simulink model "Multibody_Street_Drone"  (R2019b)
settings: Solver=FixedStepAuto  StartTime=0.0  StopTime=20  FixedStep=0.0075  MaxStep=1e-1  MinStep=1e-7  RelTol=1e-3  AbsTol=1e-6
values from neighbouring files (symbols this model uses):
  Rear_brake = [0 1.82218650851 3.8277518469 5.98774429698 7.94202318038 9.84492098434 11.9533431061 13.8561462856 16.0160441112 18.021704074 19.9760775819 21.9303564653 ... (72 elements, 36x2)]    [Rear_brake.mat]
  TPS_0 = [469.425704648 608.284708657 814.443475346 1022.3060335 1213.13067704 1420.75786613 1608.14616582 1820.50021131 2024.31741075 2213.1951296 2423.41496358 2611.22557668 ... (88 elements, 44x2)]    [TPS_0.mat]
undefined symbols (not defined in the file or in its folder): Front_brake, sigbuilder_block, X, Y, Z
libraries: sm_lib x290, nesl_utility x136, simulink x2
(part 1 of 12)
settings Model: Creator=prave  LastModifiedBy=prave
settings SolverCC: AutoScaleAbsTol=off  MaxConsecutiveMinStep=2  ZeroCrossAlgorithm=Adaptive  AlgebraicLoopSolver=LineSearch
settings DataIOCC: ReturnWorkspaceOutputs=off
settings DebuggingCC: IgnoredZcDiagnostic=none

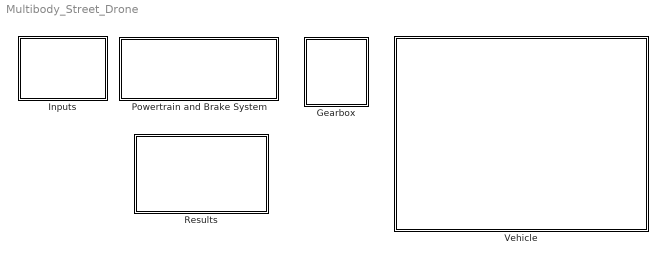
== system Multibody_Street_Drone ==
  Gearbox : Subsystem
  Inputs : Subsystem
  Powertrain and Brake System : Subsystem
  Results : Subsystem
  Vehicle : Subsystem

== system Multibody_Street_Drone/Gearbox ==
  For_reverse : Gain  Gain=-1
  Manual Switch1 : ManualSwitch  CurrentSetting=0
  Manual Switch2 : ManualSwitch
  Neutral : Constant  Value=0
  tag scope: tau=global
  wires:
  Manual Switch1/1 -> [tau]
  Neutral/1 -> Manual Switch1/1
  [final_tau] -> For_reverse/1, Manual Switch2/1
  Manual Switch2/1 -> Manual Switch1/2
  For_reverse/1 -> Manual Switch2/2

== system Multibody_Street_Drone/Inputs ==
  Delta : Subsystem
  Velocity : Subsystem

== system Multibody_Street_Drone/Powertrain and Brake System ==
  Abs : Abs
  Brake_system : Subsystem
  Divide : Product  Inputs=/*
  Driveline_viscous_losses : Subsystem
  Driver : simulink/Continuous/PID Controller  Controller=PID  Form=Parallel  TimeDomain=Continuous-time  SampleTime=-1  IntegratorMethod=Forward Euler  FilterMethod=Forward Euler  ControllerParametersSource=internal  P=150  I=1  D=0  UseFilter=on  N=100  TunerSelectOption=Transfer Function Based (PID Tuner App)  InitialConditionSource=internal  InitialConditionForIntegrator=0  InitialConditionForFilter=0  DifferentiatorICPrevScaledInput=0  ExternalReset=none  TrackingMode=off  Kt=1  LimitOutput=off  UpperSaturationLimit=inf  LowerSaturationLimit=-inf  LinearizeAsGain=on  AntiWindupMode=none  Kb=1  POutMin=[]  POutMax=[]  IOutMin=[]  IOutMax=[]  DOutMin=[]  DOutMax=[]  NOutMin=[]  NOutMax=[]  SumOutMin=[]  SumOutMax=[]  SaturationOutMin=[]  SaturationOutMax=[]  PParamMin=[]  PParamMax=[]  IParamMin=[]  IParamMax=[]  DParamMin=[]  DParamMax=[]  NParamMin=[]  NParamMax=[]  KbParamMin=[]  KbParamMax=[]  KtParamMin=[]  KtParamMax=[]  KbOutMin=[]  KbOutMax=[]  KtOutMin=[]  KtOutMax=[]  IntegratorOutMin=[]  IntegratorOutMax=[]  FilterOutMin=[]  FilterOutMax=[]  SumI1OutMin=[]  SumI1OutMax=[]  SumI2OutMin=[]  SumI2OutMax=[]  SumI3OutMin=[]  SumI3OutMax=[]  SumI4OutMin=[]  SumI4OutMax=[]  SumDOutMin=[]  SumDOutMax=[]  DifferentiatorOutMin=[]  DifferentiatorOutMax=[]  FilterDiffOutCoefMin=[]  FilterDiffOutCoefMax=[]  ReciprocalOutMin=[]  ReciprocalOutMax=[]  SumDenOutMin=[]  SumDenOutMax=[]  SumNumOutMin=[]  SumNumOutMax=[]  DivideOutMin=[]  DivideOutMax=[]  IntegratorContinuousStateAttributes=''  IntegratorStateMustResolveToSignalObject=off  IntegratorRTWStateStorageClass=Auto  FilterContinuousStateAttributes=''  FilterStateMustResolveToSignalObject=off  FilterRTWStateStorageClass=Auto  ParallelPVariant=InternalParameters  IdealPVariant=Disabled  IVariant=InternalParameters  DVariant=InternalParameters  IntegratorVariant=Continuous  SatVariant=Disabled  AWVariant=Passthrough  PCopyVariant=Disabled  TRVariant=Disabled  FdbkBlocksVariant=Forward  IdealPFdbkVariant=Disabled  SatFdbkVariant=Disabled  DerivativeFilterVariant=ContFilter  NVariant=InternalParameters  NCopyVariant=Disabled  FilterICVariant=InternalICsFilter  IntegratorICVariant=InternalICs  ExternalResetVariant=Disabled  TRSumVariant=Passthrough  SumFdbkVariant=Disabled  SumVariant=Sum_PID
  Gain1 : Gain  Gain=0.5
  Gear_ratio : Gain  Gain=9.23
  Motor : Subsystem
  Rate Limiter6 : RateLimiter  RisingSlewLimit=600  FallingSlewLimit=-1000  SampleTimeMode=inherited
  Scaling : Subsystem
  Scope : Scope
  Scope18 : Scope  NumInputPorts=2
  Subtract : Sum  Inputs=+-
  Subtract2 : Sum  Inputs=+-
  To Workspace : ToWorkspace  VariableName=Desired_Vel  SampleTime=-1
  To Workspace1 : ToWorkspace  VariableName=Motor_force  SampleTime=-1
  tag scope: Me_Pt=global, final_tau=global
  wires:
  Subtract/1 -> Driver/1  "Error"
  [Inputs] -> To Workspace/1, Scope18/1, Subtract/1  "Desired"
  Driver/1 -> Motor/2(I/p1), Brake_system/1(I/p)
  [Vel] -> Abs/1
  Motor/1(O/p) -> Subtract2/1
  Driveline_viscous_losses/1(O/p) -> Subtract2/2
  Subtract2/1 -> Gear_ratio/1
  Gear_ratio/1 -> Scaling/1(I/p)
  Scaling/1(O/p) -> Gain1/1
  [RL_Re] -> Divide/1
  Divide/1 -> To Workspace1/1
  Gain1/1 -> Rate Limiter6/1
  Abs/1 -> Motor/1(I/p2), Subtract/2, Scope18/2  "Actual"
  Rate Limiter6/1 -> [final_tau], Scope/1, Divide/2, [Me_Pt]

== system Multibody_Street_Drone/Results ==
  Actual brake torque : Subsystem
  Ay&Yaw : Subsystem
  Coordinates : Subsystem
  Fx : Subsystem
  Fy : Subsystem
  Fz : Subsystem
  Steering_angle : Subsystem
  Subsystem1 : Subsystem
  Velocity&Ax : Subsystem

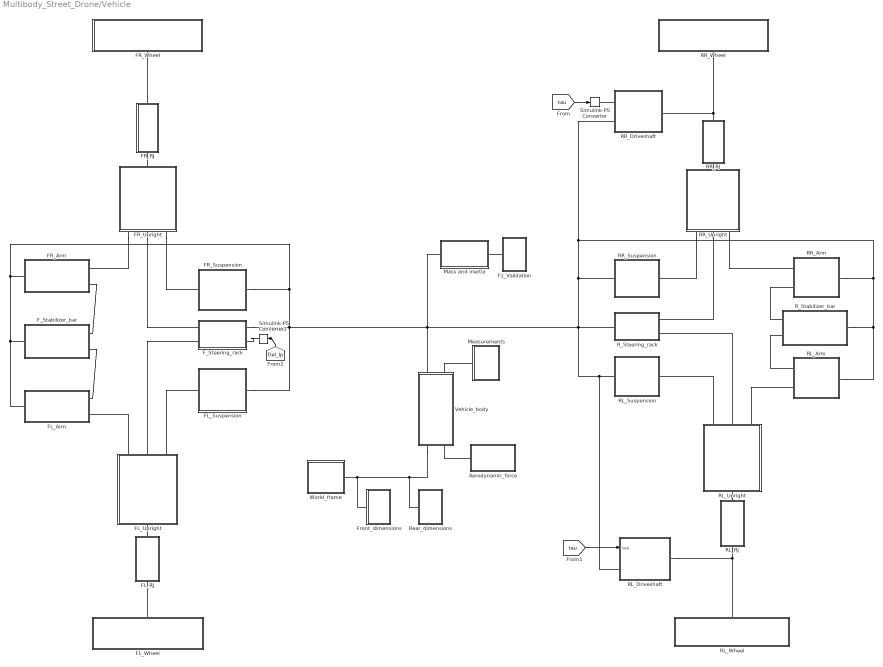
== system Multibody_Street_Drone/Vehicle ==
  Aerodynamic_force : Subsystem
  FL_Arm : Subsystem
  FL_RJ : Subsystem
  FL_Suspension : Subsystem
  FL_Upright : Subsystem
  FL_Wheel : Subsystem
  FR_Arm : Subsystem
  FR_RJ : Subsystem
  FR_Suspension : Subsystem
  FR_Upright : Subsystem
  FR_Wheel : Subsystem
  F_Stabilizer_bar : Subsystem
  F_Steering_rack : Subsystem
  Front_dimensions : Subsystem
  Fz_Validation : Subsystem
  Mass and inertia : Subsystem
  Measurements : Subsystem
  RL_Arm : Subsystem
  RL_Driveshaft : Subsystem
  RL_RJ : Subsystem
  RL_Suspension : Subsystem
  RL_Upright : Subsystem
  RL_Wheel : Subsystem
  RR_Arm : Subsystem
  RR_Driveshaft : Subsystem
  RR_RJ : Subsystem
  RR_Suspension : Subsystem
  RR_Upright : Subsystem
  RR_Wheel : Subsystem
  R_Stabilizer_bar : Subsystem
  R_Steering_rack : Subsystem
  Rear_dimensions : Subsystem
  Simulink-PS Converter : nesl_utility/Simulink-PS Converter  PhysicalDomain=network_engine_domain  SubClassName=ps_input  LeftPortType=input  RightPortType=output  PseudoPeriodic=off  Frequencies=[]  NoiseDistribution=none  NoiseParameters=[]  Unit=1  AffineConversion=off  FilteringAndDerivatives=provide  SimscapeFilterOrder=1  InputFilterTimeConstant=0.001  UdotUserProvided=0
  Simulink-PS Converter2 : nesl_utility/Simulink-PS Converter  PhysicalDomain=network_engine_domain  SubClassName=ps_input  LeftPortType=input  RightPortType=output  PseudoPeriodic=off  Frequencies=[]  NoiseDistribution=none  NoiseParameters=[]  Unit=cm  AffineConversion=off  FilteringAndDerivatives=filter  SimscapeFilterOrder=2  InputFilterTimeConstant=0.001  UdotUserProvided=0
  Vehicle_body : Subsystem
  World_frame : Subsystem
  wires:
  [tau] -> Simulink-PS Converter/1
  [Del_Ip] -> Simulink-PS Converter2/1
  [tau] -> RL_Driveshaft/1(tau)
  connections:
  RL_Arm/RConn1 -- R_Stabilizer_bar/RConn2
  FL_Upright/LConn3 -- FL_Suspension/RConn1
  F_Stabilizer_bar/RConn2 -- FL_Arm/RConn1
  FL_Upright/LConn1 -- FL_Arm/RConn2
  Simulink-PS Converter2/RConn1 -- F_Steering_rack/LConn2
  R_Stabilizer_bar/RConn1 -- RR_Arm/RConn2
  RL_Upright/RConn2 -- R_Steering_rack/RConn2
  FR_Upright/LConn3 -- FR_Suspension/RConn1
  FL_Arm/LConn1 -- F_Stabilizer_bar/LConn1 -- FR_Arm/LConn1 -- FR_Suspension/LConn1 -- F_Steering_rack/LConn1 -- FL_Suspension/LConn1 -- Mass and inertia/LConn1 -- RL_Driveshaft/LConn1 -- RL_Suspension/LConn1 -- R_Steering_rack/LConn1 -- RR_Driveshaft/LConn2 -- R_Stabilizer_bar/LConn1 -- RL_Arm/LConn1 -- RR_Arm/LConn1 -- RR_Suspension/LConn1 -- Vehicle_body/LConn1
  RR_Upright/LConn2 -- R_Steering_rack/RConn1
  RL_Upright/RConn3 -- RL_Arm/RConn2
  FL_Upright/LConn2 -- F_Steering_rack/RConn2
  FR_RJ/LConn1 -- FR_Upright/RConn1
  RR_Upright/LConn3 -- RR_Arm/RConn1
  FR_Upright/LConn2 -- F_Steering_rack/RConn1
  RR_Upright/LConn1 -- RR_Suspension/RConn1
  RL_Upright/RConn1 -- RL_Suspension/RConn1
  FL_Upright/RConn1 -- FL_RJ/LConn1
  Vehicle_body/RConn1 -- Rear_dimensions/LConn1 -- Front_dimensions/LConn1 -- World_frame/RConn1
  Measurements/RConn1 -- Vehicle_body/LConn2
  RL_Upright/LConn1 -- RL_RJ/LConn1
  RR_Driveshaft/LConn1 -- Simulink-PS Converter/RConn1
  RR_Upright/RConn1 -- RR_RJ/LConn1
  FR_Upright/LConn1 -- FR_Arm/RConn1
  Aerodynamic_force/LConn1 -- Vehicle_body/RConn2
  FR_Arm/RConn2 -- F_Stabilizer_bar/RConn1
  FR_RJ/RConn1 -- FR_Wheel/LConn1
  FL_Wheel/LConn1 -- FL_RJ/RConn1
  RL_Driveshaft/RConn1 -- RL_Wheel/LConn1 -- RL_RJ/RConn1
  RR_Driveshaft/RConn1 -- RR_Wheel/LConn1 -- RR_RJ/RConn1
  Fz_Validation/LConn1 -- Mass and inertia/RConn1

== system Multibody_Street_Drone/Inputs/Delta ==
  Constant2 : Constant  Value=0
  Del : Subsystem  Tag=STV Subsys  LoadFcn=sigbuilder_block('load');  StartFcn=sigbuilder_block('start');  StopFcn=sigbuilder_block('stop');  ClipboardFcn=sigbuilder_block('clipboard');  mask(Sigbuilder block){tuvar=[0:10]}
      mask help: Simulink:masks:SigbuilderBlock_MD
      mask init:
      | if ~strcmp(get_param(bdroot(gcbh),'SimulationStatus'),'stopped') tuvar = sigbuilder_block('maskInit'); end
      settings: CopyFcn=sigbuilder_block('copy');  DeleteFcn=sigbuilder_block('delete');  ModelCloseFcn=sigbuilder_block('modelClose');  PreSaveFcn=sigbuilder_block('preSave');  PauseFcn=sigbuilder_block('pause');  ContinueFcn=sigbuilder_block('continue');  NameChangeFcn=sigbuilder_block('namechange');  OpenFcn=sigbuilder_block('open',[5.4 72.6 1141.2 513.6 ]);  CloseFcn=sigbuilder_block('close');
      mask Display: plot(0, 0, 100, 100,[2, 2, 32, 32, 2], [68, 8, 8, 68, 68],[32, 2], [38, 38], [32, 19, 2],[53, 60, 44], [32, 17, 17, 2],[16, 16, 31, 31]);txt = getActiveGroup(gcbh);text(2, 100, txt,'verticalAlignment', 'top');
  Manual Switch3 : ManualSwitch  CurrentSetting=0
  Radius_of_pinion_cms : Gain  Gain=0.56
  Scope1 : Scope
  To Workspace : ToWorkspace  VariableName=del_hand_wheel  SampleTime=-1
  to_radians : Gain  Gain=pi/180
  tag scope: Del_Ip=global, Del_Ip_hand=global
  wires:
  Radius_of_pinion_cms/1 -> to_radians/1
  Constant2/1 -> Manual Switch3/1
  to_radians/1 -> Manual Switch3/2
  Manual Switch3/1 -> Scope1/1, [Del_Ip]
  Del/1(Signal 1) -> To Workspace/1, [Del_Ip_hand], Radius_of_pinion_cms/1

== system Multibody_Street_Drone/Inputs/Velocity ==
  Forward : Subsystem  Tag=STV Subsys  LoadFcn=sigbuilder_block('load');  StartFcn=sigbuilder_block('start');  StopFcn=sigbuilder_block('stop');  ClipboardFcn=sigbuilder_block('clipboard');  mask(Sigbuilder block){tuvar=[0:10]}
      mask help: Simulink:masks:SigbuilderBlock_MD
      mask init:
      | if ~strcmp(get_param(bdroot(gcbh),'SimulationStatus'),'stopped') tuvar = sigbuilder_block('maskInit'); end
      settings: CopyFcn=sigbuilder_block('copy');  DeleteFcn=sigbuilder_block('delete');  ModelCloseFcn=sigbuilder_block('modelClose');  PreSaveFcn=sigbuilder_block('preSave');  PauseFcn=sigbuilder_block('pause');  ContinueFcn=sigbuilder_block('continue');  NameChangeFcn=sigbuilder_block('namechange');  OpenFcn=sigbuilder_block('open',[5.4 0 1141.2 552.6 ]);  CloseFcn=sigbuilder_block('close');
      mask Display: plot(0, 0, 100, 100,[2, 2, 32, 32, 2], [68, 8, 8, 68, 68],[32, 2], [38, 38], [32, 19, 2],[53, 60, 44], [32, 17, 17, 2],[16, 16, 31, 31]);txt = getActiveGroup(gcbh);text(2, 100, txt,'verticalAlignment', 'top');
  Manual Switch1 : ManualSwitch
  Reverse : Subsystem  Tag=STV Subsys  LoadFcn=sigbuilder_block('load');  StartFcn=sigbuilder_block('start');  StopFcn=sigbuilder_block('stop');  ClipboardFcn=sigbuilder_block('clipboard');  mask(Sigbuilder block){tuvar=[0:10]}
      mask help: Simulink:masks:SigbuilderBlock_MD
      mask init:
      | if ~strcmp(get_param(bdroot(gcbh),'SimulationStatus'),'stopped') tuvar = sigbuilder_block('maskInit'); end
      settings: CopyFcn=sigbuilder_block('copy');  DeleteFcn=sigbuilder_block('delete');  ModelCloseFcn=sigbuilder_block('modelClose');  PreSaveFcn=sigbuilder_block('preSave');  PauseFcn=sigbuilder_block('pause');  ContinueFcn=sigbuilder_block('continue');  NameChangeFcn=sigbuilder_block('namechange');  OpenFcn=sigbuilder_block('open',[5.4 0 1141.2 552.6 ]);  CloseFcn=sigbuilder_block('close');
      mask Display: plot(0, 0, 100, 100,[2, 2, 32, 32, 2], [68, 8, 8, 68, 68],[32, 2], [38, 38], [32, 19, 2],[53, 60, 44], [32, 17, 17, 2],[16, 16, 31, 31]);txt = getActiveGroup(gcbh);text(2, 100, txt,'verticalAlignment', 'top');
  tag scope: Inputs=global
  wires:
  Manual Switch1/1 -> [Inputs]
  Forward/1(Signal 1) -> Manual Switch1/1
  Reverse/1(Signal 1) -> Manual Switch1/2

== system Multibody_Street_Drone/Powertrain and Brake System/Brake_system ==
  I/p : Inport
  Brake_pedal : Saturate  UpperLimit=0  LowerLimit=-100
  Front_brake : Lookup_n-D  NumberOfTableDimensions=1  BreakpointsForDimension1=[Front_brake(:,1)]  Table=[Front_brake(:,2)]  InternalRulePriority=Speed  RndMeth=Simplest  InputSameDT=on
  Gain1 : Gain  Gain=-1
  Gain11 : Gain  Gain=-1/100
  Gain2 : Gain  Gain=0.5
  Gain3 : Gain  Gain=0.5
  Max_Br_pr : Gain  Gain=71.7
  Rear_brake : Lookup_n-D  NumberOfTableDimensions=1  BreakpointsForDimension1=[Rear_brake(:,1)]  Table=[Rear_brake(:,2)]  InternalRulePriority=Speed  RndMeth=Simplest  InputSameDT=on
  Scope{25,28..29,31} (4 alike) : Scope
  To Workspace1 : ToWorkspace  VariableName=brake_pr  SampleTime=-1
  To Workspace2 : ToWorkspace  VariableName=brake_pedal  SampleTime=-1
  tag scope: brTau_F=global, brTau_R=global, br_pedal=global
  wires:
  Gain1/1 -> [br_pedal], To Workspace2/1
  I/p/1 -> Brake_pedal/1
  Brake_pedal/1 -> Gain11/1, Scope29/1
  Gain11/1 -> Max_Br_pr/1, Gain1/1
  Front_brake/1 -> Gain2/1, Scope25/1
  Rear_brake/1 -> Gain3/1, Scope28/1
  Max_Br_pr/1 -> Rear_brake/1, Scope31/1, To Workspace1/1, Front_brake/1
  Gain2/1 -> [brTau_F]
  Gain3/1 -> [brTau_R]

== system Multibody_Street_Drone/Powertrain and Brake System/Driveline_viscous_losses ==
  Gain : Gain  Gain=-1
  Product : Product
  Scope : Scope
  Scope1 : Scope
  Switch : Switch
  Viscous_friction1 : Gain  Commented=on  Gain=2
  Viscous_friction2 : Gain  Gain=2.537
  O/p : Outport
  tag scope: PT_loss=global
  wires:
  [Vel] -> Viscous_friction2/1
  Viscous_friction2/1 -> [PT_loss], Scope1/1, Product/1
  [RL_Re] -> Product/2
  Product/1 -> Gain/1, Switch/1
  Switch/1 -> Scope/1, O/p/1
  Gain/1 -> Switch/3
  [motor_tau] -> Switch/2

== system Multibody_Street_Drone/Powertrain and Brake System/Motor ==
  I/p2 : Inport
  I/p1 : Inport  Port=2
  % : Gain  Gain=1/100
  %1 : Gain  Gain=100
  2-D Lookup Table2 : Lookup_n-D  BreakpointsForDimension1=[0 0.1 0.2 0.3 0.4 0.5 0.6 0.7 0.8 0.9 1]  BreakpointsForDimension2=[TPS_0(:,1)]  Table=[-90.24,-90.26,-90.24,-90.22,-90.23,-86.63,-72.71,-56.25,-50.21,-44.59,-40.69,-37.61,-34.44,-31.97,-29.79,-27.98,-26.37,-24.7,-23.15,-22.11,-21.24,-20.43,-19.47,-18.66,-17.94,-17.25,-16.58,-15.87,-15.16,-14.33,-14.11,-14.27,-14.21,-13.57,-12.89,-12.82,-12.72,-12.45,-12.19,-11.94,-11.65,-11.38,-10.97,-10.65;-25.48,-25.71,-26.16,-26.77,-27.52,-28.39,-29.45,-30.61,-30.61,-30.63,-30.66,-30.57,-29.83,-28.1,-26.6,-25.1,-23.88,-22.46,-21.12,-19.91,-18.49,-17.4,-16.44,-15.32,-14.29,-13.12,-11.74,-10.25,-9.37,-8.72,-8.56,-8.89,-9.14,-8.69,-8.35,-8.5,-8.76,-8.73,-8.69,-8.74,-8.78,-8.93,-8.85,-8.81;-3.28,-3.05,-2.62,-2.39,-2.44,-2.48,-2.54,-2.68,-2.6,-2.61,-2.62,-2.68,-2.68,-2.82,-2.75,-2.82,-2.8,-2.89,-2.94,-2.63,-2.34,-2.19,-2.46,-2.64,-2.54,-2.48,-2.51,-2.49,-2.26,-2.06,-2.09,-2.06,-2.16,-2.2,-2.19,-2.17,-2.12,-2.11,-2.09,-2.23,-2.18,-2.22,-1.91,-1.71;1.59,1.32,0.82,0.49,0.72,0.7,0.69,0.55,0.55,0.52,0.54,0.5,0.5,0.39,0.41,0.36,0.38,0.23,0.01,0.14,0.44,0.56,0.42,0.38,0.4,0.46,0.52,0.71,0.75,0.99,0.75,0.46,0.17,0.45,0.71,0.69,0.65,0.71,0.82,0.8,0.7,0.73,0.91,0.92;5.53,5.09,4.45,4.29,4.5,4.55,4.53,4.39,4.32,4.22,4.1,4.06,4.01,3.82,3.78,3.79,3.8,3.5,3.19,3.26,3.52,3.61,3.6,3.59,3.55,3.57,3.62,3.78,3.97,3.97,3.63,3.07,2.54,3,3.46,3.3,3.14,3.1,3.27,3.29,3.3,3.06,2.88,2.84;11.33,11.26,11.2,11.21,10.97,10.69,10.7,10.72,10.6,10.38,10.35,10.42,10.44,10.4,10.37,10.44,10.42,10.2,9.95,9.89,9.91,10,10.21,10.45,10.54,10.47,10.24,10,9.95,9.95,9.53,8.87,8.33,8.47,8.53,8.42,8.17,7.92,7.49,6.94,6.33,5.85,5.3,4.85;19.11,19.06,18.77,18.67,18.7,18.8,18.81,18.68,18.55,18.37,18.27,18.37,18.48,18.55,18.66,18.83,18.83,18.34,17.79,17.71,17.81,17.64,17.34,17.04,16.9,16.68,15.98,15.04,14.42,13.6,13.18,13.07,12.52,11.53,10.55,9.6,8.86,8.15,7.54,6.96,6.32,5.82,5.24,4.81;28.1,27.9,27.6,27.49,27.67,27.85,27.84,27.8,27.76,27.77,27.76,27.84,28.04,28.6,28.91,28.63,28.44,27.35,26.18,25.07,23.8,22.59,21.41,20.1,18.89,17.45,16.55,15.16,14.38,13.65,13.21,13.12,12.81,11.71,10.47,9.58,8.86,8.18,7.49,6.88,6.29,5.83,5.28,4.83;38.54,38.36,38.01,37.97,37.85,37.92,38.01,37.99,38.11,38.21,38.5,38.77,38.13,36.15,34.04,31.71,29.64,28.1,26.66,25.34,23.91,22.61,21.39,19.98,18.93,17.7,16.64,15.08,14.25,13.64,13.12,13.07,12.71,11.68,10.8,9.77,9.04,8.19,7.49,6.92,6.31,5.83,5.31,4.83;48.94,48.7,48.33,48.29,48.4,48.63,48.94,49.25,48.39,47.53,45.18,42.6,39.77,37.17,34.71,32.24,30.04,28.31,26.94,25.48,23.97,22.66,21.47,20.21,18.88,17.9,16.58,15.05,14.15,13.52,13.13,13.14,12.85,11.73,10.81,9.85,8.99,8.18,7.54,6.97,6.28,5.79,5.32,4.87;63.83,63.82,63.58,63.85,64.53,63.91,59.28,54.29,52.51,49.2,46.19,43.52,40.41,37.58,35.15,32.9,30.85,29.41,28.22,26.87,25.46,24.15,22.97,21.67,20.45,19.12,17.73,16.37,15.59,15.04,14.59,14.63,14.39,13.51,12.63,11.73,11.04,10.31,9.81,9.23,8.67,8.26,7.72,7.31]  InternalRulePriority=Speed  RndMeth=Simplest  InputSameDT=on
  2-D Lookup Table5 : Lookup_n-D  BreakpointsForDimension1=[0.3 0.4 0.5 0.6 0.7 0.8 0.9 1]  BreakpointsForDimension2=[TPS_0(:,1)]  Table=[1.59,1.32,0.82,0.49,0.72,0.7,0.69,0.55,0.55,0.52,0.54,0.5,0.5,0.39,0.41,0.36,0.38,0.23,0.01,0.14,0.44,0.56,0.42,0.38,0.4,0.46,0.52,0.71,0.75,0.99,0.75,0.46,0.17,0.45,0.71,0.69,0.65,0.71,0.82,0.8,0.7,0.73,0.91,0.92;5.53,5.09,4.45,4.29,4.5,4.55,4.53,4.39,4.32,4.22,4.1,4.06,4.01,3.82,3.78,3.79,3.8,3.5,3.19,3.26,3.52,3.61,3.6,3.59,3.55,3.57,3.62,3.78,3.97,3.97,3.63,3.07,2.54,3,3.46,3.3,3.14,3.1,3.27,3.29,3.3,3.06,2.88,2.84;11.33,11.26,11.2,11.21,10.97,10.69,10.7,10.72,10.6,10.38,10.35,10.42,10.44,10.4,10.37,10.44,10.42,10.2,9.95,9.89,9.91,10,10.21,10.45,10.54,10.47,10.24,10,9.95,9.95,9.53,8.87,8.33,8.47,8.53,8.42,8.17,7.92,7.49,6.94,6.33,5.85,5.3,4.85;19.11,19.06,18.77,18.67,18.7,18.8,18.81,18.68,18.55,18.37,18.27,18.37,18.48,18.55,18.66,18.83,18.83,18.34,17.79,17.71,17.81,17.64,17.34,17.04,16.9,16.68,15.98,15.04,14.42,13.6,13.18,13.07,12.52,11.53,10.55,9.6,8.86,8.15,7.54,6.96,6.32,5.82,5.24,4.81;28.1,27.9,27.6,27.49,27.67,27.85,27.84,27.8,27.76,27.77,27.76,27.84,28.04,28.6,28.91,28.63,28.44,27.35,26.18,25.07,23.8,22.59,21.41,20.1,18.89,17.45,16.55,15.16,14.38,13.65,13.21,13.12,12.81,11.71,10.47,9.58,8.86,8.18,7.49,6.88,6.29,5.83,5.28,4.83;38.54,38.36,38.01,37.97,37.85,37.92,38.01,37.99,38.11,38.21,38.5,38.77,38.13,36.15,34.04,31.71,29.64,28.1,26.66,25.34,23.91,22.61,21.39,19.98,18.93,17.7,16.64,15.08,14.25,13.64,13.12,13.07,12.71,11.68,10.8,9.77,9.04,8.19,7.49,6.92,6.31,5.83,5.31,4.83;48.94,48.7,48.33,48.29,48.4,48.63,48.94,49.25,48.39,47.53,45.18,42.6,39.77,37.17,34.71,32.24,30.04,28.31,26.94,25.48,23.97,22.66,21.47,20.21,18.88,17.9,16.58,15.05,14.15,13.52,13.13,13.14,12.85,11.73,10.81,9.85,8.99,8.18,7.54,6.97,6.28,5.79,5.32,4.87;63.83,63.82,63.58,63.85,64.53,63.91,59.28,54.29,52.51,49.2,46.19,43.52,40.41,37.58,35.15,32.9,30.85,29.41,28.22,26.87,25.46,24.15,22.97,21.67,20.45,19.12,17.73,16.37,15.59,15.04,14.59,14.63,14.39,13.51,12.63,11.73,11.04,10.31,9.81,9.23,8.67,8.26,7.72,7.31]  InternalRulePriority=Speed  RndMeth=Simplest  InputSameDT=on
  Derivative : Derivative
  Motor_rpm : Subsystem
  Saturation : Saturate  UpperLimit=1  LowerLimit=0.19
  Scope{,2,14,16,26,30,32} (7 alike) : Scope
  Switch : Switch  Criteria=u2 ~= 0
  Throttle : Saturate  UpperLimit=100  LowerLimit=0
  To Workspace : ToWorkspace  VariableName=tau  SampleTime=-1
  To Workspace1 : ToWorkspace  VariableName=throttle  SampleTime=-1
  condition_for_regen : simulink/Logic and Bit Operations/Compare To Constant  relop=>=  const=1  OutDataTypeStr=boolean
  O/p : Outport
  tag scope: motor_tau=global
  wires:
  I/p2/1 -> condition_for_regen/1
  %/1 -> Scope32/1, Saturation/1, 2-D Lookup Table2/1, %1/1
  Motor_rpm/1(Out1) -> 2-D Lookup Table5/2, 2-D Lookup Table2/2
  2-D Lookup Table5/1 -> Switch/3, Scope14/1
  condition_for_regen/1 -> Switch/2, Scope2/1
  Saturation/1 -> 2-D Lookup Table5/1
  2-D Lookup Table2/1 -> Switch/1, Scope30/1
  Switch/1 -> [motor_tau], To Workspace/1, Derivative/1, Scope16/1, O/p/1
  I/p1/1 -> Throttle/1
  Derivative/1 -> Scope/1
  %1/1 -> To Workspace1/1, Scope26/1
  Throttle/1 -> %/1

== system Multibody_Street_Drone/Powertrain and Brake System/Scaling ==
  I/p : Inport
  Constant : Constant  Value=112.3
  Motor_gain : Gain  Gain=1.086
  Product : Product
  Scope : Scope
  Scope1 : Scope
  Subtract2 : Sum
  O/p : Outport
  tag scope: Before_gear=global
  wires:
  Motor_gain/1 -> Scope1/1, Subtract2/1
  Subtract2/1 -> [Before_gear], O/p/1
  I/p/1 -> Motor_gain/1
  Constant/1 -> Product/1
  [RL_Re] -> Product/2
  Product/1 -> Subtract2/2, Scope/1

== system Multibody_Street_Drone/Results/Actual brake torque ==
  Add : Sum
  Add1 : Sum
  To Workspace : ToWorkspace  VariableName=brTau_F  SampleTime=-1
  To Workspace2 : ToWorkspace  VariableName=brTau_R  SampleTime=-1
  wires:
  Add/1 -> To Workspace/1
  [act_br_FL] -> Add/1
  [act_br_FR] -> Add/2
  [act_br_RR] -> Add1/2
  [act_br_RL] -> Add1/1
  Add1/1 -> To Workspace2/1

== system Multibody_Street_Drone/Results/Ay&Yaw ==
  Divide4 : Product  Inputs=*/
  To Workspace1 : ToWorkspace  VariableName=Yaw  SampleTime=-1
  To Workspace4 : ToWorkspace  VariableName=ay  SampleTime=-1
  wires:
  [Fy_total] -> Divide4/1
  Divide4/1 -> To Workspace4/1
  [mass] -> Divide4/2
  [Yaw_rate] -> To Workspace1/1

== system Multibody_Street_Drone/Results/Coordinates ==
  To Workspace2 : ToWorkspace  VariableName=Y_SD  SampleTime=-1
  To Workspace8 : ToWorkspace  VariableName=X_SD  SampleTime=-1
  wires:
  [X] -> To Workspace8/1
  [Y] -> To Workspace2/1

== system Multibody_Street_Drone/Results/Fx ==
  Actual : Subsystem
  Calculated : Subsystem

== system Multibody_Street_Drone/Results/Fy ==
  Add3 : Sum  Inputs=++++
  Add4 : Sum
  Add5 : Sum
  Gain3 : Gain  Gain=-1
  To Workspace : ToWorkspace  VariableName=Fy_front  SampleTime=-1
  To Workspace1 : ToWorkspace  VariableName=Fy_rear  SampleTime=-1
  To Workspace10 : ToWorkspace  VariableName=actual_Fy_vehicle  SampleTime=-1
  To Workspace11 : ToWorkspace  VariableName=actual_Fy_RL  SampleTime=-1
  To Workspace12 : ToWorkspace  VariableName=actual_Fy_RR  SampleTime=-1
  tag scope: Fy_F=global, Fy_R=global, Fy_total=global
  wires:
  Add5/1 -> [Fy_R], To Workspace1/1
  Add4/1 -> [Fy_F], To Workspace/1
  Add3/1 -> To Workspace10/1, [Fy_total]
  [FR_Fy] -> Add4/2, Add3/2
  [RR_Fy] -> Gain3/1
  Gain3/1 -> To Workspace12/1, Add5/2, Add3/4
  [RL_Fy] -> Add5/1, To Workspace11/1, Add3/3
  [FL_Fy] -> Add3/1, Add4/1

== system Multibody_Street_Drone/Results/Fz ==
  Plot Tire Results : Subsystem
      settings: OpenFcn=PlotTireOutputs_UI
      mask Display: disp('Plot Tire Results');
  Sensing : Subsystem
  Tire Forces : Scope
  wires:
  Sensing/1(Fz) -> Tire Forces/1

== system Multibody_Street_Drone/Results/Steering_angle ==
  Constant : Constant  Value=0.01683
  Gain : Gain  Gain=0.5
  Gain1 : Gain  Gain=180/pi
  Gain2 : Gain  Gain=180/pi
  Gain3 : Gain  Gain=180/pi
  Subtract : Sum  Inputs=+-
  Subtract1 : Sum
  Subtract2 : Sum
  To Workspace1 : ToWorkspace  VariableName=del_road_wheel  SampleTime=-1
  To Workspace15 : ToWorkspace  VariableName=Del  SampleTime=-1
  To Workspace2 : ToWorkspace  VariableName=del_road_wheel_L  SampleTime=-1
  To Workspace3 : ToWorkspace  VariableName=del_road_wheel_R  SampleTime=-1
  tag scope: Del_Act_Ang=global, Del_Op=global
  wires:
  Gain1/1 -> To Workspace1/1, [Del_Act_Ang]
  Subtract2/1 -> Gain/1
  Constant/1 -> Subtract/2, Subtract1/1
  Subtract/1 -> Subtract2/1, Gain2/1
  [Del_R] -> Subtract1/2
  Subtract1/1 -> Subtract2/2, Gain3/1
  [Del_L] -> Subtract/1
  Gain/1 -> To Workspace15/1, [Del_Op], Gain1/1
  Gain2/1 -> To Workspace2/1
  Gain3/1 -> To Workspace3/1

== system Multibody_Street_Drone/Results/Subsystem1 ==
  Add : Sum
  Add1 : Sum  Inputs=++++
  Add2 : Sum
  Gain : Gain  Gain=0.0151
  To Workspace : ToWorkspace  VariableName=Drag_force  SampleTime=-1
  To Workspace1 : ToWorkspace  VariableName=Total_long_force  SampleTime=-1
  tag scope: Drag_force=global, Total_long_force=global
  wires:
  [Aero_loss] -> Add1/2
  [PT_loss] -> Add1/1
  [Fz_total] -> Gain/1
  [Iner_loss_L] -> Add/1
  [Iner_loss_R] -> Add/2
  Add/1 -> Add1/4
  Add1/1 -> To Workspace/1, [Drag_force], Add2/1
  [Fx] -> Add2/2
  Add2/1 -> [Total_long_force], To Workspace1/1
  Gain/1 -> Add1/3

== system Multibody_Street_Drone/Results/Velocity&Ax ==
  Add1 : Sum  Inputs=++++
  Derivative : Derivative
  Gain : Gain  Gain=-1
  Gain9 : Gain  Gain=0.25
  Scope3 : Scope  NumInputPorts=4
  To Workspace1 : ToWorkspace  VariableName=Actual_Vel  SampleTime=-1
  To Workspace2 : ToWorkspace  VariableName=Act_Ax  SampleTime=-1
  tag scope: Act_Ax=global, Vel=global
  wires:
  Add1/1 -> Gain9/1
  Gain/1 -> Scope3/4, Add1/4
  [FR_Vx] -> Scope3/2, Add1/2
  [RL_Vx] -> Scope3/3, Add1/3
  [RR_Vx] -> Gain/1
  [FL_Vx] -> Scope3/1, Add1/1
  Derivative/1 -> To Workspace2/1, [Act_Ax]
  Gain9/1 -> [Vel], To Workspace1/1, Derivative/1

== system Multibody_Street_Drone/Vehicle/Aerodynamic_force ==
  External Force and Torque : sm_lib/Forces and Torques/External Force and Torque  ForceResolutionFrame=AttachedFrame  EnableForceX=on  EnableForceY=off  EnableForceZ=off  EnableForce=off  TorqueResolutionFrame=AttachedFrame  EnableTorqueX=off  EnableTorqueY=off  EnableTorqueZ=off  EnableTorque=off
  Gain : Gain  Gain=0.5
  Product : Product  Inputs=3
  Rigid Transform : sm_lib/Frames and Transforms/Rigid Transform  TranslationMethod=Cartesian  TranslationStandardOffset=1.169  TranslationLengthUnit=m  TranslationStandardAxis=+X  TranslationCartesianOffset=[1.169 0 -0.1305]  TranslationROffset=0  TranslationROffsetUnits=m  TranslationZOffset=0  TranslationZOffsetUnits=m  TranslationThetaOffset=0  TranslationThetaOffsetUnits=deg  RotationMethod=StandardAxis  RotationAngleUnits=deg  RotationStandardAxis=+Z  RotationAngle=180  RotationArbitraryAxis=[0 0 1]  FollAlignAxisA=+X  BaseAlignAxisA=+Y  FollAlignAxisB=+Y  BaseAlignAxisB=+Z  RotationSequenceAxes=FollowerAxes  RotationSequence=XYX  RotationSequenceAngles=[0 0 0]  RotationSequenceAnglesUnits=deg  RotationMatrix=[1 0 0; 0 1 0; 0 0 1]
  Scope : Scope
  Simulink-PS Converter3 : nesl_utility/Simulink-PS Converter  PhysicalDomain=network_engine_domain  SubClassName=ps_input  LeftPortType=input  RightPortType=output  PseudoPeriodic=off  Frequencies=[]  NoiseDistribution=none  NoiseParameters=[]  Unit=1  AffineConversion=off  FilteringAndDerivatives=provide  SimscapeFilterOrder=1  InputFilterTimeConstant=0.001  UdotUserProvided=0
  row*SCx : Constant  Value=0.81
  row*SCx1 : Constant  Value=0.804288
  vehicle_body : PMIOPort  Side=Left
  tag scope: Aero_loss=global
  wires:
  row*SCx1/1 -> Product/1
  Gain/1 -> [Aero_loss], Scope/1, Simulink-PS Converter3/1
  [Vel] -> Product/3
  [Vel] -> Product/2
  Product/1 -> Gain/1
  connections:
  Rigid Transform/LConn1 -- vehicle_body/RConn1
  Simulink-PS Converter3/RConn1 -- External Force and Torque/LConn1
  Rigid Transform/RConn1 -- External Force and Torque/RConn1

== system Multibody_Street_Drone/Vehicle/FL_Arm ==
  FL arm : sm_lib/Body Elements/Extruded Solid  GraphicAmbientColor=[0.15 0.15 0.15 1.0]  BasedOnType=Mass  CenterOfMass=[0 0 0]  CenterOfMassUnits=m  GraphicDiffuseColor=[0.5 0.5 0.5]  ExtrusionCrossSection=[10 14.471; -10 14.471; -10 -14.471; 10 -14.471]  ExtrusionCrossSectionUnits=cm  Density=1000  DensityUnits=kg/m^3  DoExposeReferenceFrame=off  GraphicEmissiveColor=[0.0 0.0 0.0 1.0]  ExportEntireGeometry=off  ExtrusionLength=1  ExtrusionLengthUnits=cm  ExtrusionType=General  SerializedFrames=<Frames><Frame><Id>Frame1</Id><Value><Name>F1</Name><Origin><Source>GeometricFeature</Source><FeatureName>side surface 3</FeatureName></Origin><PrimaryAxis><DefinedDirection>+X</DefinedDirection><Source>ReferenceFrame</Source><SourceDirection>+Z</SourceDirection><FeatureName></FeatureName></PrimaryAxis><SecondaryAxis><DefinedDirection>+Y</DefinedDirection><Source>ReferenceFrame</Source><SourceDirection>+Y</SourceDirection><FeatureName></FeatureName></SecondaryAxis></Value></Frame><Frame><Id>Frame2</Id><Value><Name>F2</Name><Origin><Source>GeometricFeature</Source><FeatureName>side surface 1</FeatureName></Origin><PrimaryAxis><DefinedDirection>+Z</DefinedDirection><Source>ReferenceFrame</Source><SourceDirection>+Y</SourceDirection><FeatureName></FeatureName></PrimaryAxis><SecondaryAxis><DefinedDirection>+Y</DefinedDirection><Source>ReferenceFrame</Source><SourceDirection>+X</SourceDirection><FeatureName></FeatureName></SecondaryAxis></Value></Frame></Frames>  MarkerShape=Sphere  MarkerSize=10  GraphicType=FromGeometry  InertiaType=CalculateFromGeometry  Mass=3  MassUnits=kg  MomentsOfInertia=[1 1 1]  MomentsOfInertiaUnits=kg*m^2  PolygonNumSides=3  GraphicOpacity=1.0  PolygonOuterRadius=1  PolygonOuterRadiusUnits=m  ProductsOfInertia=[0 0 0]  ProductsOfInertiaUnits=kg*m^2  GraphicShininess=75  GraphicSpecularColor=[0.5 0.5 0.5 1.0]  GraphicVisPropType=SimpleVisualProperties
  Revolute Joint : sm_lib/Joints/Revolute Joint  JointMode=Normal  SenseConstraintForce=off  SenseConstraintForceX=off  SenseConstraintForceY=off  SenseConstraintForceZ=off  SenseConstraintTorque=off  SenseConstraintTorqueX=off  SenseConstraintTorqueY=off  SenseConstraintTorqueZ=off  SenseTotalForce=off  SenseTotalForceX=off  SenseTotalForceY=off  SenseTotalForceZ=off  SenseTotalTorque=off  SenseTotalTorqueX=off  SenseTotalTorqueY=off  SenseTotalTorqueZ=off  CompositeWrenchDir=FollowerOnBase  CompositeWrenchFrame=BaseFrame  EquilibriumPosition=0  EquilibriumPositionUnits=deg  SpringStiffness=0  SpringStiffnessUnits=N*m/deg  DampingCoefficient=0  DampingCoefficientUnits=N*m/(deg/s)  TorqueActuationMode=NoTorque  MotionActuationMode=ComputedMotion  SensePosition=off  SenseVelocity=off  SenseAcceleration=off  SenseTorqueForce=off  SenseLowerLimitTorqueForce=off  SenseUpperLimitTorqueForce=off  LowerLimitSpecify=off  LowerLimitBound=-90  LowerLimitBoundUnits=deg  LowerLimitStiffness=1e4  LowerLimitStiffnessUnits=N*m/deg  LowerLimitDamping=10  LowerLimitDampingUnits=N*m/(deg/s)  LowerLimitTransitionRegionWidth=0.1  LowerLimitTransitionRegionWidthUnits=deg  UpperLimitSpecify=off  UpperLimitBound=90  UpperLimitBoundUnits=deg  UpperLimitStiffness=1e4  UpperLimitStiffnessUnits=N*m/deg  UpperLimitDamping=10  UpperLimitDampingUnits=N*m/(deg/s)  UpperLimitTransitionRegionWidth=0.1  UpperLimitTransitionRegionWidthUnits=deg  PositionTargetSpecify=off  PositionTargetPriority=High  PositionTargetValue=0  PositionTargetValueUnits=deg  VelocityTargetSpecify=off  VelocityTargetPriority=High  VelocityTargetValue=0  VelocityTargetValueUnits=deg/s
  Rigid Transform1 : sm_lib/Frames and Transforms/Rigid Transform  TranslationMethod=Cartesian  TranslationStandardOffset=0  TranslationLengthUnit=m  TranslationStandardAxis=+Z  TranslationCartesianOffset=[0.03625 -0.08055 -0.0027]  TranslationROffset=0  TranslationROffsetUnits=m  TranslationZOffset=0  TranslationZOffsetUnits=m  TranslationThetaOffset=0  TranslationThetaOffsetUnits=deg  RotationMethod=None  RotationAngleUnits=deg  RotationStandardAxis=+Z  RotationAngle=0.0  RotationArbitraryAxis=[0 0 1]  FollAlignAxisA=+X  BaseAlignAxisA=-Y  FollAlignAxisB=+Y  BaseAlignAxisB=+Z  RotationSequenceAxes=FollowerAxes  RotationSequence=XYX  RotationSequenceAngles=[0 0 0]  RotationSequenceAnglesUnits=deg  RotationMatrix=[1 0 0; 0 1 0; 0 0 1]
  Rigid Transform13 : sm_lib/Frames and Transforms/Rigid Transform  TranslationMethod=None  TranslationStandardOffset=0  TranslationLengthUnit=m  TranslationStandardAxis=+Z  TranslationCartesianOffset=[0.0377 0.08337 -0.1277]  TranslationROffset=0  TranslationROffsetUnits=m  TranslationZOffset=0  TranslationZOffsetUnits=m  TranslationThetaOffset=0  TranslationThetaOffsetUnits=deg  RotationMethod=AlignedAxes  RotationAngleUnits=deg  RotationStandardAxis=+Z  RotationAngle=0.0  RotationArbitraryAxis=[0 0 1]  FollAlignAxisA=+X  BaseAlignAxisA=-Y  FollAlignAxisB=+Y  BaseAlignAxisB=+Z  RotationSequenceAxes=FollowerAxes  RotationSequence=XYX  RotationSequenceAngles=[0 0 0]  RotationSequenceAnglesUnits=deg  RotationMatrix=[1 0 0; 0 1 0; 0 0 1]
  Rigid Transform7 : sm_lib/Frames and Transforms/Rigid Transform  TranslationMethod=Cartesian  TranslationStandardOffset=0  TranslationLengthUnit=m  TranslationStandardAxis=+Z  TranslationCartesianOffset=[0.97281 0.17335 -0.27437]  TranslationROffset=0  TranslationROffsetUnits=m  TranslationZOffset=0  TranslationZOffsetUnits=m  TranslationThetaOffset=0  TranslationThetaOffsetUnits=deg  RotationMethod=None  RotationAngleUnits=deg  RotationStandardAxis=+Z  RotationAngle=0.0  RotationArbitraryAxis=[0 0 1]  FollAlignAxisA=+X  BaseAlignAxisA=+Y  FollAlignAxisB=+Y  BaseAlignAxisB=+Z  RotationSequenceAxes=FollowerAxes  RotationSequence=XYX  RotationSequenceAngles=[0 0 0]  RotationSequenceAnglesUnits=deg  RotationMatrix=[1 0 0; 0 1 0; 0 0 1]
  Rigid Transform8 : sm_lib/Frames and Transforms/Rigid Transform  TranslationMethod=None  TranslationStandardOffset=0  TranslationLengthUnit=m  TranslationStandardAxis=+Z  TranslationCartesianOffset=[0.9728 0.173 -0.274]  TranslationROffset=0  TranslationROffsetUnits=m  TranslationZOffset=0  TranslationZOffsetUnits=m  TranslationThetaOffset=0  TranslationThetaOffsetUnits=deg  RotationMethod=StandardAxis  RotationAngleUnits=deg  RotationStandardAxis=+Y  RotationAngle=90  RotationArbitraryAxis=[0 0 1]  FollAlignAxisA=+X  BaseAlignAxisA=+Y  FollAlignAxisB=+Y  BaseAlignAxisB=+Z  RotationSequenceAxes=FollowerAxes  RotationSequence=XYX  RotationSequenceAngles=[0 0 0]  RotationSequenceAnglesUnits=deg  RotationMatrix=[1 0 0; 0 1 0; 0 0 1]
  Spherical Joint1 : sm_lib/Joints/Spherical Joint  JointMode=Normal  SenseConstraintForce=off  SenseConstraintForceX=off  SenseConstraintForceY=off  SenseConstraintForceZ=off  SenseConstraintTorque=off  SenseConstraintTorqueX=off  SenseConstraintTorqueY=off  SenseConstraintTorqueZ=off  SenseTotalForce=off  SenseTotalForceX=off  SenseTotalForceY=off  SenseTotalForceZ=off  SenseTotalTorque=off  SenseTotalTorqueX=off  SenseTotalTorqueY=off  SenseTotalTorqueZ=off  CompositeWrenchDir=FollowerOnBase  CompositeWrenchFrame=BaseFrame  DefPosRotationMethod=None  DefPosRotationAngleUnits=deg  DefPosRotationStandardAxis=+Z  DefPosRotationAngle=0.0  DefPosRotationArbitraryAxis=[0 0 1]  DefPosFollAlignAxisA=+X  DefPosBaseAlignAxisA=+Y  DefPosFollAlignAxisB=+Y  DefPosBaseAlignAxisB=+Z  DefPosRotationSequenceAxes=FollowerAxes  DefPosRotationSequence=XYX  DefPosRotationSequenceAngles=[0 0 0]  DefPosRotationSequenceAnglesUnits=deg  DefPosRotationMatrix=[1 0 0; 0 1 0; 0 0 1]  EqPosRotationMethod=None  EqPosRotationAngleUnits=deg  EqPosRotationStandardAxis=+Z  EqPosRotationAngle=0.0  EqPosRotationArbitraryAxis=[0 0 1]  EqPosFollAlignAxisA=+X  EqPosBaseAlignAxisA=+Y  EqPosFollAlignAxisB=+Y  EqPosBaseAlignAxisB=+Z  EqPosRotationSequenceAxes=FollowerAxes  EqPosRotationSequence=XYX  EqPosRotationSequenceAngles=[0 0 0]  EqPosRotationSequenceAnglesUnits=deg  EqPosRotationMatrix=[1 0 0; 0 1 0; 0 0 1]  SpringStiffness=0  SpringStiffnessUnits=N*m/deg  DampingCoefficient=0  DampingCoefficientUnits=N*m/(deg/s)  ActuateTorqueX=on  ActuateTorqueY=on  ActuateTorqueZ=on  ActuateTorque=off  TorqueActuationMode=NoTorque  MotionActuationMode=ComputedMotion  ActuationFrame=BaseFrame  SensePosition=off  SenseVelocityX=off  SenseVelocityY=off  SenseVelocityZ=off  SenseVelocity=off  SenseAccelerationX=off  SenseAccelerationY=off  SenseAccelerationZ=off  SenseAcceleration=off  SenseTorqueX=off  SenseTorqueY=off  SenseTorqueZ=off  SenseTorqueForce=off  SenseLowerLimitTorqueMag=off  SenseUpperLimitTorqueMag=off  SensingFrame=BaseFrame  LowerLimitSpecify=off  LowerLimitBound=15  LowerLimitBoundUnits=deg  LowerLimitStiffness=1e4  LowerLimitStiffnessUnits=N*m/deg  LowerLimitDamping=10  LowerLimitDampingUnits=N*m/(deg/s)  LowerLimitTransitionRegionWidth=0.1  LowerLimitTransitionRegionWidthUnits=deg  UpperLimitSpecify=off  UpperLimitBound=45  UpperLimitBoundUnits=deg  UpperLimitStiffness=1e4  UpperLimitStiffnessUnits=N*m/deg  UpperLimitDamping=10  UpperLimitDampingUnits=N*m/(deg/s)  UpperLimitTransitionRegionWidth=0.1  UpperLimitTransitionRegionWidthUnits=deg  PositionTargetRotationMethod=None  PositionTargetRotationAngleUnits=deg  PositionTargetRotationStandardAxis=+Z  PositionTargetRotationAngle=0.0  PositionTargetRotationArbitraryAxis=[0 0 1]  PositionTargetFollAlignAxisA=+X  PositionTargetBaseAlignAxisA=+Y  PositionTargetFollAlignAxisB=+Y  PositionTargetBaseAlignAxisB=+Z  PositionTargetRotationSequenceAxes=FollowerAxes  PositionTargetRotationSequence=XYX  PositionTargetRotationSequenceAngles=[0 0 0]  PositionTargetRotationSequenceAnglesUnits=deg  PositionTargetRotationMatrix=[1 0 0; 0 1 0; 0 0 1]  PositionTargetSpecify=off  PositionTargetPriority=High  VelocityTargetValue=[0 0 0]  VelocityTargetValueUnits=deg/s  VelocityTargetSpecify=off  VelocityTargetPriority=Low  VelocityTargetInFollowerFrame=off
  chassis : PMIOPort  Side=Left
  stabilizer_bar : PMIOPort  Port=2  Side=Right
  upright : PMIOPort  Port=3  Side=Right
  connections:
  FL arm/RConn1 -- Rigid Transform13/LConn1
  FL arm/LConn1 -- Revolute Joint/RConn1
  Rigid Transform8/RConn1 -- Revolute Joint/LConn1
  Rigid Transform8/LConn1 -- Rigid Transform7/RConn1
  Rigid Transform13/RConn1 -- Rigid Transform1/LConn1 -- Spherical Joint1/LConn1
  Rigid Transform7/LConn1 -- chassis/RConn1
  upright/RConn1 -- Spherical Joint1/RConn1
  Rigid Transform1/RConn1 -- stabilizer_bar/RConn1

== system Multibody_Street_Drone/Vehicle/FL_RJ ==
  Gain : Gain  Gain=-1
  PS-Simulink Converter : nesl_utility/PS-Simulink Converter  PhysicalDomain=network_engine_domain  SubClassName=ps_output  LeftPortType=input  RightPortType=output  PseudoPeriodic=off  Frequencies=[]  Unit=inherit  AffineConversion=off
  PS-Simulink Converter1 : nesl_utility/PS-Simulink Converter  PhysicalDomain=network_engine_domain  SubClassName=ps_output  LeftPortType=input  RightPortType=output  PseudoPeriodic=off  Frequencies=[]  Unit=inherit  AffineConversion=off
  PS-Simulink Converter2 : nesl_utility/PS-Simulink Converter  PhysicalDomain=network_engine_domain  SubClassName=ps_output  LeftPortType=input  RightPortType=output  PseudoPeriodic=off  Frequencies=[]  Unit=inherit  AffineConversion=off
  RJ_FL : sm_lib/Joints/Revolute Joint  JointMode=Normal  SenseConstraintForce=off  SenseConstraintForceX=off  SenseConstraintForceY=off  SenseConstraintForceZ=off  SenseConstraintTorque=off  SenseConstraintTorqueX=off  SenseConstraintTorqueY=off  SenseConstraintTorqueZ=off  SenseTotalForce=off  SenseTotalForceX=off  SenseTotalForceY=off  SenseTotalForceZ=off  SenseTotalTorque=off  SenseTotalTorqueX=off  SenseTotalTorqueY=off  SenseTotalTorqueZ=off  CompositeWrenchDir=FollowerOnBase  CompositeWrenchFrame=BaseFrame  EquilibriumPosition=0  EquilibriumPositionUnits=deg  SpringStiffness=0  SpringStiffnessUnits=N*m/deg  DampingCoefficient=0  DampingCoefficientUnits=N*m/(deg/s)  TorqueActuationMode=InputTorque  MotionActuationMode=ComputedMotion  SensePosition=off  SenseVelocity=on  SenseAcceleration=on  SenseTorqueForce=on  SenseLowerLimitTorqueForce=off  SenseUpperLimitTorqueForce=off  LowerLimitSpecify=off  LowerLimitBound=-90  LowerLimitBoundUnits=deg  LowerLimitStiffness=1e4  LowerLimitStiffnessUnits=N*m/deg  LowerLimitDamping=10  LowerLimitDampingUnits=N*m/(deg/s)  LowerLimitTransitionRegionWidth=0.1  LowerLimitTransitionRegionWidthUnits=deg  UpperLimitSpecify=off  UpperLimitBound=90  UpperLimitBoundUnits=deg  UpperLimitStiffness=1e4  UpperLimitStiffnessUnits=N*m/deg  UpperLimitDamping=10  UpperLimitDampingUnits=N*m/(deg/s)  UpperLimitTransitionRegionWidth=0.1  UpperLimitTransitionRegionWidthUnits=deg  PositionTargetSpecify=off  PositionTargetPriority=High  PositionTargetValue=0  PositionTargetValueUnits=deg  VelocityTargetSpecify=off  VelocityTargetPriority=High  VelocityTargetValue=52.39  VelocityTargetValueUnits=rad/s
  Rigid Transform2 : sm_lib/Frames and Transforms/Rigid Transform  TranslationMethod=StandardAxis  TranslationStandardOffset=4  TranslationLengthUnit=cm  TranslationStandardAxis=+Z  TranslationCartesianOffset=[0 0 0]  TranslationROffset=0  TranslationROffsetUnits=m  TranslationZOffset=0  TranslationZOffsetUnits=m  TranslationThetaOffset=0  TranslationThetaOffsetUnits=deg  RotationMethod=None  RotationAngleUnits=deg  RotationStandardAxis=+Z  RotationAngle=0.0  RotationArbitraryAxis=[0 0 1]  FollAlignAxisA=+X  BaseAlignAxisA=+Y  FollAlignAxisB=+Y  BaseAlignAxisB=+Z  RotationSequenceAxes=FollowerAxes  RotationSequence=XYX  RotationSequenceAngles=[0 0 0]  RotationSequenceAnglesUnits=deg  RotationMatrix=[1 0 0; 0 1 0; 0 0 1]
  Scope : Scope  NumInputPorts=3
  Scope1 : Scope
  Simulink-PS Converter : nesl_utility/Simulink-PS Converter  PhysicalDomain=network_engine_domain  SubClassName=ps_input  LeftPortType=input  RightPortType=output  PseudoPeriodic=off  Frequencies=[]  NoiseDistribution=none  NoiseParameters=[]  Unit=1  AffineConversion=off  FilteringAndDerivatives=provide  SimscapeFilterOrder=1  InputFilterTimeConstant=0.001  UdotUserProvided=0
  Switch : Switch  Criteria=u2 > Threshold
  upright : PMIOPort  Side=Left
  wheel : PMIOPort  Port=2  Side=Right
  tag scope: act_br_FL=global
  wires:
  PS-Simulink Converter/1 -> Scope/1
  PS-Simulink Converter1/1 -> Scope/2
  PS-Simulink Converter2/1 -> [act_br_FL], Scope/3
  Switch/1 -> Scope1/1, Simulink-PS Converter/1
  Gain/1 -> Switch/3
  [Vel] -> Switch/2
  [brTau_F] -> Gain/1, Switch/1
  connections:
  wheel/RConn1 -- Rigid Transform2/LConn1
  RJ_FL/LConn1 -- upright/RConn1
  PS-Simulink Converter/LConn1 -- RJ_FL/RConn2
  PS-Simulink Converter1/LConn1 -- RJ_FL/RConn3
  PS-Simulink Converter2/LConn1 -- RJ_FL/RConn4
  Simulink-PS Converter/RConn1 -- RJ_FL/LConn2
  Rigid Transform2/RConn1 -- RJ_FL/RConn1
